simulink model "PNG_guidanceloop_errorAnalysis_19b"  (R2019b)
settings: Solver=VariableStepAuto  StartTime=0.0  StopTime=15  RelTol=1e-3
values from neighbouring files (symbols this model uses):
  aT = 1    [errSlxParas.m]
  coeffs_den = double(fliplr(coeffs(eq_den,s)))    [errSlxParas.m]
  coeffs_num = double(fliplr(coeffs(eq_num,s)))    [errSlxParas.m]
  epi = 1    [errSlxParas.m]
  phiGN = 1    [errSlxParas.m]
  Tf = 1    [errSlxParas.m]
  Tf_Tg = 15    [errSlxParas.m]
  Tg = 1    [errSlxParas.m]
  Vm = 1    [errSlxParas.m]
settings Model: OrderedModelArguments=off  Creator=anwaei  LastModifiedBy=anwaei

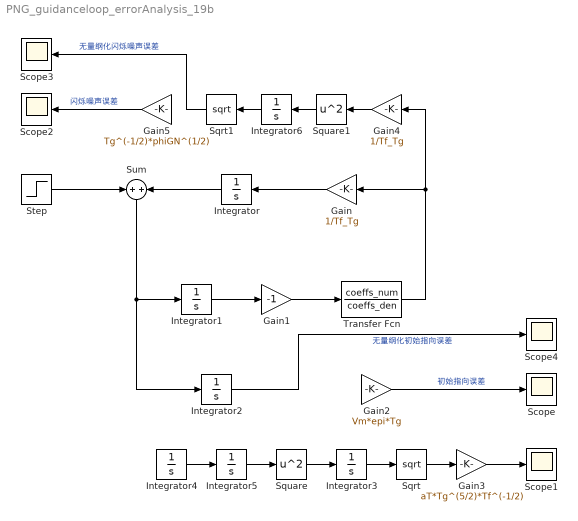
== system PNG_guidanceloop_errorAnalysis_19b ==
  Gain : Gain  Gain=1/Tf_Tg
  Gain1 : Gain  Gain=-1
  Gain2 : Gain  Gain=Vm*epi*Tg
  Gain3 : Gain  Gain=aT*Tg^(5/2)*Tf^(-1/2)
  Gain4 : Gain  Gain=1/Tf_Tg
  Gain5 : Gain  Gain=Tg^(-1/2)*phiGN^(1/2)
  Integrator{,1..6} (7 alike) : Integrator
  Scope{,1..4} (5 alike) : Scope
  Sqrt : Sqrt  SaturateOnIntegerOverflow=on
  Sqrt1 : Sqrt  SaturateOnIntegerOverflow=on
  Square : Math  Operator=square  SaturateOnIntegerOverflow=on
  Square1 : Math  Operator=square  SaturateOnIntegerOverflow=on
  Step : Step  SampleTime=0
  Sum : Sum  Inputs=+|+
  Transfer Fcn : TransferFcn  Numerator=coeffs_num  Denominator=coeffs_den
  wires:
  Step/1 -> Sum/1
  Integrator/1 -> Sum/2
  Gain/1 -> Integrator/1
  Integrator4/1 -> Integrator5/1
  Sum/1 -> Integrator1/1, Integrator2/1
  Integrator2/1 -> Scope4/1  "无量纲化初始指向误差"
  Integrator1/1 -> Gain1/1
  Gain1/1 -> Transfer Fcn/1
  Transfer Fcn/1 -> Gain4/1, Gain/1
  Gain4/1 -> Square1/1
  Square1/1 -> Integrator6/1
  Integrator6/1 -> Sqrt1/1
  Sqrt1/1 -> Scope3/1  "无量纲化闪烁噪声误差"
  Integrator5/1 -> Square/1
  Square/1 -> Integrator3/1
  Integrator3/1 -> Sqrt/1
  Sqrt/1 -> Gain3/1
  Gain5/1 -> Scope2/1  "闪烁噪声误差"
  Gain2/1 -> Scope/1  "初始指向误差"
  Gain3/1 -> Scope1/1
